simulink model "engine_with_auto_transmission_4spd_crcr"  (R2026a)
settings: Solver=VariableStepAuto  StopTime=15
libraries: nesl_utility x16, fl_lib x12, sdl_lib x9
settings Model: Creator=doyeop  LastModifiedBy=doyeop

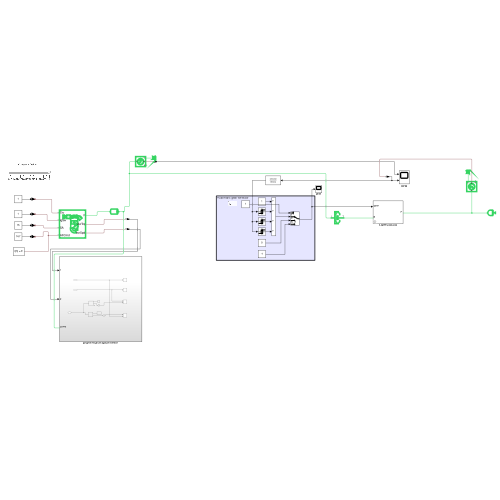
[thumbnail: Simulink's stored preview of the top-level diagram]
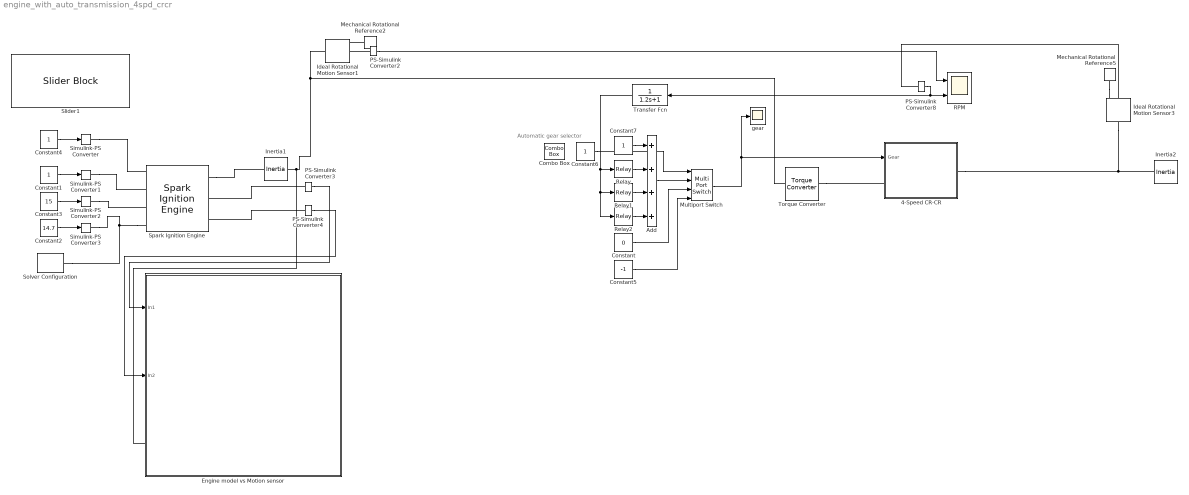
== system engine_with_auto_transmission_4spd_crcr ==
  note: Automatic gear selector
  4-Speed CR-CR : Subsystem  mask(4-Speed CR-CR){InitGear=Neutral, ShowInLibBrowser=0, ClutchSchedule={[0 1 1 0 0];[1 1 0 0 0];[1 0 1 0 0];[1 0 0 1 0];[0 0 0 1 1];[0 0 0 1 0]}}
      mask prompts: InitGear "Initial gear"
      mask help: physmod:sdl:library:transmissions:FourSpeedCRCR
      mask init:
      | set_param([gcb,'/Clutch A'],'initial_state_locked',num2str(ClutchSchedule{InitGear}(1)));
      | set_param([gcb,'/Clutch B'],'initial_state_locked',num2str(ClutchSchedule{InitGear}(2)));
      | set_param([gcb,'/Clutch C'],'initial_state_locked',num2str(ClutchSchedule{InitGear}(3)));
      | set_param([gcb,'/Clutch D'],'initial_state_locked',num2str(ClutchSchedule{InitGear}(4)));
      | set_param([gcb,'/Clutch R'],'initial_state_locked',num2str(ClutchSchedule{InitGear}(5)));
      mask Help: web([docroot '/sdl/ref/4speedcrcr.html'])
      mask TypeOptions InitGear: 4 | 3 | 2 | 1 | physmod:sdl:library:transmissions:Reverse | physmod:sdl:library:transmissions:Neutral
  Add : Sum  Inputs=++++
  Combo Box : ComboBox  LabelPosition=Hide  SelectedLabel=D
  Constant : Constant  Value=0
  Constant1 : Constant
  Constant2 : Constant  Value=14.7  SampleTime=-1
  Constant3 : Constant  Value=15  SampleTime=-1
  Constant4 : Constant  SampleTime=-1
  Constant5 : Constant  Value=-1
  Constant6 : Constant
  Constant7 : Constant
  Engine model vs Motion sensor : Subsystem
  Ideal Rotational Motion Sensor1 : fl_lib/Mechanical/Mechanical Sensors/Ideal Rotational Motion Sensor  reference=foundation.enum.MeasurementReference.difference  acceleration_port=false  velocity_port=true  position_port=true  wrap_angle=false  offset=0 rad
  Ideal Rotational Motion Sensor3 : fl_lib/Mechanical/Mechanical Sensors/Ideal Rotational Motion Sensor  reference=foundation.enum.MeasurementReference.difference  acceleration_port=false  velocity_port=true  position_port=true  wrap_angle=false  offset=0 rad
  Inertia1 : fl_lib/Mechanical/Rotational Elements/Inertia  inertia=0.7 kg*m^2  num_ports=foundation.enum.numPorts2.two  w_specify=on  w_priority=High  w=1200 rpm  w_nominal_specify=off  w_nominal_value=1  w_nominal_unit=rad/s  t_specify=off  t_priority=None  t=0 N*m  t_nominal_specify=off  t_nominal_value=1  t_nominal_unit=N*m
  Inertia2 : fl_lib/Mechanical/Rotational Elements/Inertia  inertia=0.5 kg*m^2  num_ports=foundation.enum.numPorts2.one  w_specify=on  w_priority=None  w=0 rpm  w_nominal_specify=off  w_nominal_value=1  w_nominal_unit=rad/s  t_specify=off  t_priority=None  t=0 N*m  t_nominal_specify=off  t_nominal_value=1  t_nominal_unit=N*m
  Mechanical Rotational Reference2 : fl_lib/Mechanical/Rotational Elements/Mechanical Rotational Reference
  Mechanical Rotational Reference5 : fl_lib/Mechanical/Rotational Elements/Mechanical Rotational Reference
  Multiport Switch : MultiPortSwitch  DataPortOrder=Specify indices  DataPortIndices={1,0,-1}  SaturateOnIntegerOverflow=off  InputSameDT=off
  PS-Simulink Converter2 : nesl_utility/PS-Simulink Converter  PhysicalDomain=network_engine_domain  SubClassName=ps_output  LeftPortType=input  RightPortType=output  PseudoPeriodic=off  Frequencies=[]  VectorFormat=inherit  Unit=rpm  AffineConversion=off
  PS-Simulink Converter3 : nesl_utility/PS-Simulink Converter  PhysicalDomain=network_engine_domain  SubClassName=ps_output  LeftPortType=input  RightPortType=output  PseudoPeriodic=off  Frequencies=[]  VectorFormat=inherit  Unit=N*m  AffineConversion=off
  PS-Simulink Converter4 : nesl_utility/PS-Simulink Converter  PhysicalDomain=network_engine_domain  SubClassName=ps_output  LeftPortType=input  RightPortType=output  PseudoPeriodic=off  Frequencies=[]  VectorFormat=inherit  Unit=rpm  AffineConversion=off
  PS-Simulink Converter8 : nesl_utility/PS-Simulink Converter  PhysicalDomain=network_engine_domain  SubClassName=ps_output  LeftPortType=input  RightPortType=output  PseudoPeriodic=off  Frequencies=[]  VectorFormat=inherit  Unit=rpm  AffineConversion=off
  RPM : Scope  NumInputPorts=2
      settings: ActiveDisplayYMinimum=-326.02351905011483  ActiveDisplayYMaximum=2934.21167144869  DataLoggingVariableName=ScopeData3
  Relay : Relay  OnSwitchValue=500  OffSwitchValue=300
  Relay1 : Relay  OnSwitchValue=750  OffSwitchValue=500
  Relay2 : Relay  OnSwitchValue=1500  OffSwitchValue=750
  Simulink-PS Converter : nesl_utility/Simulink-PS Converter  PhysicalDomain=network_engine_domain  SubClassName=ps_input  LeftPortType=input  RightPortType=output  PseudoPeriodic=off  Frequencies=[]  NoiseDistribution=none  NoiseParameters=[]  Unit=1  AffineConversion=off  FilteringAndDerivatives=provide  SimscapeFilterOrder=1  InputFilterTimeConstant=0.001  UdotUserProvided=0
  Simulink-PS Converter1 : nesl_utility/Simulink-PS Converter  PhysicalDomain=network_engine_domain  SubClassName=ps_input  LeftPortType=input  RightPortType=output  PseudoPeriodic=off  Frequencies=[]  NoiseDistribution=none  NoiseParameters=[]  Unit=1  AffineConversion=off  FilteringAndDerivatives=provide  SimscapeFilterOrder=1  InputFilterTimeConstant=0.001  UdotUserProvided=0
  Simulink-PS Converter2 : nesl_utility/Simulink-PS Converter  PhysicalDomain=network_engine_domain  SubClassName=ps_input  LeftPortType=input  RightPortType=output  PseudoPeriodic=off  Frequencies=[]  NoiseDistribution=none  NoiseParameters=[]  Unit=deg  AffineConversion=off  FilteringAndDerivatives=provide  SimscapeFilterOrder=1  InputFilterTimeConstant=0.001  UdotUserProvided=0
  Simulink-PS Converter3 : nesl_utility/Simulink-PS Converter  PhysicalDomain=network_engine_domain  SubClassName=ps_input  LeftPortType=input  RightPortType=output  PseudoPeriodic=off  Frequencies=[]  NoiseDistribution=none  NoiseParameters=[]  Unit=1  AffineConversion=off  FilteringAndDerivatives=provide  SimscapeFilterOrder=1  InputFilterTimeConstant=0.001  UdotUserProvided=0
  Slider1 : SliderBlock  ScaleMax=1
  Solver Configuration : nesl_utility/Solver Configuration  PhysicalDomain=network_engine_domain  SubClassName=solver  LeftPortType=input  RightPortType=generic  Tones=[]  Harmonics=[]  SimulateNoise=off  Profile=off  UseLocalSampling=off  EnableSwitchedLinearOptims=on  FrequencyDomain=off  UseCCode=off  RelTol=0.001  AbsTol=0.001  MinStep=1e-09  ToWorkspace=off  RevertToSquareIcSolve=off  NumHomotopyIterations=100  PhasorMode=off  PhasorModeNumHarmonics=1  ConsistencySolver=NEWTON_XTOL_AFTER_FTOL  CanonicalOrdering=CANONICAL  OptimizeIntermediates=OPTIMIZED  IndexReductionMethod=DerivativeReplacement  DoDC=off  ResidualTolerance=1e-09  ConsistencyTolSource=GLOBAL  ConsistencyAbsTol=0.001  ConsistencyRelTol=0.001  ConsistencyTolFactor=0.001  UseLocalSolver=off  LocalSolverChoice=NE_BACKWARD_EULER_ADVANCER  ResolveIndetEquations=on  FunctionEvalNumThread=1  LocalSolverSampleTime=0.001  DoFixedCost=off  MaxNonlinIter=3  MaxModeIter=2  ComputeImpulses=off  ImpulseIterations=2  LinearAlgebra=auto  LinearAlgebraNumThread=0  EquationFormulation=NE_TIME_EF  DelaysMemoryBudget=1024  AutomaticFiltering=on  FilteringTimeConstant=0.001  PartitionStorageMethod=AS_NEEDED  PartitionMemoryBudget=1024  PartitionMethod=ROBUST  MultibodyUseLocalSolver=off  MultibodyLocalSolverChoice=ODE1  MultibodyLocalSolverSampleTime=0.001
  Spark Ignition Engine : sdl_lib/Engines & Motors/Spark Ignition Engine  numCyls=sdl.enum.engineNumCylinders.Four  twoCylSADiff=270 deg  L4FiringOrder=sdl.enum.engineFiringOrderFourCylinders.L4_1342  bore=67 mm  stroke=42.5 mm  conrod=90 mm  CR=12.2  P_amb=101.325 kPa  T_amb=298.15 K  rho_air=1.225 mg/cm^3  R_air=288.1965 J/(K*kg)  UseAirIntake=true  c_thr=0.1 s  thr_rest=3 deg  D_plate=8 cm  S_leak=0.3 cm^2  V_im=500 cm^3  Cd_in=0.9  IVO_0=-10 deg  IVC_0=100 deg  EVO_0=30 deg  EVC_0=5 deg  UseInVVT=false  UseExVVT=false  q_LHV=44.3 MJ/kg  InputAFR=true  AFR_const=14.6  InputInjPw=false  Sinj=6.5 mg/ms  SparkInputType=sdl.enum.engineSparkInputType.Angle  SA_const=20 deg  comb_bd=50 deg  dt_Pcyl_slow_decay=60 s  dt_Tcyl_slow_decay=600 s  dt_exh_decay=5 ms  InputBackPressure=false  dP_exh=50 kPa  dw_exh=6000 rpm  UseExhaustThermal=true  S_exh=1 m^2  M_exh=5 kg  C_exh=100 J/(K*kg)  k_gas=10 s  h_convection=100 W/(K*m^2)  k_radiation=0.3  SB=5.7e-8 W/(K^4*m^2)  Pim_0=101.325 kPa  ca0=0 deg  w0=0 rpm  EngSpdSimLimit=16000 rpm  OutputTorqueAvr=true  OutputSpeedAvr=true  OutputCrkpos=false  OutputPim=false  OutputAirMassFlow=false  OutputFuelMassFlow=false  OutputAFR=false  OutputVcyl=false  OutputPcyl=false  OutputTcyl=false  OutputTexh=false
  Torque Converter : sdl_lib/Couplings & Drives/Torque Converter  coast_mode_modeling=sdl.enum.torqueConverterContinuousTwomode.twomode  SR_drive_tlu=[0, .5, .6, .7, .8, .87, .92, .94, .96, .97, 1]  TR_drive_tlu=[2.232, 1.5462, 1.4058, 1.2746, 1.1528, 1.0732, 1.0192, 1, 1, 1, 1]  CF_drive_tlu=1e-4 * [.72558, .66322, .63463, .59042, .51331, .4144, .29287, .22444, .12186, .04386, 0] N*m/rpm^2  SR_coast_tlu=[0, .5, .6, .7, .8, .87, .92, .94, .96, .97, 1]  CF_coast_tlu=1e-4 * [.5079, .4643, .4442, .4133, .3593, .2901, .205, .1571, .0853, .0307, 0] N*m/rpm^2  iniMode=sdl.enum.torqueConverterInitialMode.coast  delta_w=1 rpm  n_vector=[0, .5, .6, .7, .8, .87, .92, .94, .96, .97]  trq_vector=[2.232, 1.5462, 1.4058, 1.2746, 1.1528, 1.0732, 1.0192, .9983, .9983, .9983]  cf_vector_parameterization=sdl.enum.torqueConverterCFParameterization.SpeedToSqrtTorque  cf_vector_reference_speed=sdl.enum.torqueConverterCFReferenceSpeed.ImpellerSpeedAlways  cf_vector=[12.2938, 12.8588, 13.1452, 13.6285, 14.6163, 16.2675, 19.3503, 22.1046, 29.9986, 50] rad/(N^(1/2)*m^(1/2)*s)  cf_vector_sq=1e-3 * [6.616, 6.048, 5.787, 5.384, 4.681, 3.779, 2.671, 2.047, 1.111, .4] N*m*s^2/rad^2  interp_method=simscape.enum.interpolation.linear  extrap_method=simscape.enum.extrapolation.linear  model_lag=sdl.enum.torqueConverterLagOnOff.LagOff  tau=.02 s  initial_trq_ratio=0
  Transfer Fcn : TransferFcn  Denominator=[1.2 1]
  gear : Scope
      settings: ActiveDisplayYMinimum=0.62500000000000011  ActiveDisplayYMaximum=4.375  DataLoggingVariableName=ScopeData2
  wires:
  Constant2/1 -> Simulink-PS Converter3/1
  Constant3/1 -> Simulink-PS Converter2/1
  Constant4/1 -> Simulink-PS Converter/1
  Constant1/1 -> Simulink-PS Converter1/1
  PS-Simulink Converter2/1 -> RPM/1
  PS-Simulink Converter3/1 -> Engine model vs Motion sensor/1(In1)
  PS-Simulink Converter4/1 -> Engine model vs Motion sensor/2(In2)
  PS-Simulink Converter8/1 -> RPM/2, Transfer Fcn/1
  Constant6/1 -> Multiport Switch/1
  Constant/1 -> Multiport Switch/3
  Constant5/1 -> Multiport Switch/4
  Constant7/1 -> Add/1
  Relay/1 -> Add/2
  Relay1/1 -> Add/3
  Relay2/1 -> Add/4
  Add/1 -> Multiport Switch/2
  Multiport Switch/1 -> 4-Speed CR-CR/1(Gear), gear/1
  Transfer Fcn/1 -> Relay/1, Relay1/1, Relay2/1
  connections:
  Spark Ignition Engine/LConn4 -- Simulink-PS Converter3/RConn1 -- Solver Configuration/RConn1
  Simulink-PS Converter2/RConn1 -- Spark Ignition Engine/LConn3
  Simulink-PS Converter1/RConn1 -- Spark Ignition Engine/LConn2
  PS-Simulink Converter3/LConn1 -- Spark Ignition Engine/RConn2
  Simulink-PS Converter/RConn1 -- Spark Ignition Engine/LConn1
  Spark Ignition Engine/RConn1 -- Inertia1/RConn1
  PS-Simulink Converter4/LConn1 -- Spark Ignition Engine/RConn3
  PS-Simulink Converter2/LConn1 -- Ideal Rotational Motion Sensor1/RConn2
  Mechanical Rotational Reference2/LConn1 -- Ideal Rotational Motion Sensor1/RConn1
  Ideal Rotational Motion Sensor3/RConn2 -- PS-Simulink Converter8/LConn1
  Mechanical Rotational Reference5/LConn1 -- Ideal Rotational Motion Sensor3/RConn1
  Engine model vs Motion sensor/LConn1 -- Ideal Rotational Motion Sensor1/LConn1 -- Torque Converter/LConn1 -- Inertia1/LConn1
  Ideal Rotational Motion Sensor3/LConn1 -- 4-Speed CR-CR/RConn1 -- Inertia2/LConn1
  Torque Converter/RConn1 -- 4-Speed CR-CR/LConn1

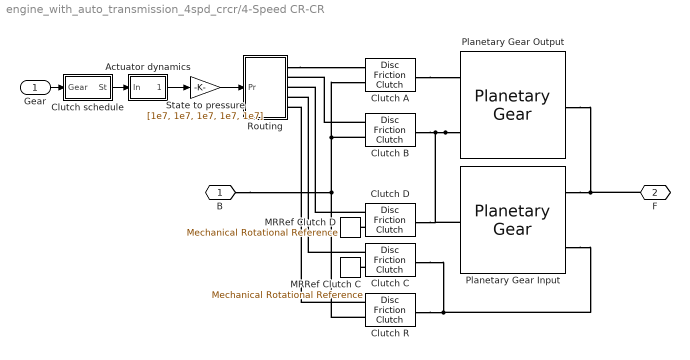
== system engine_with_auto_transmission_4spd_crcr/4-Speed CR-CR ==
  Gear : Inport
  Actuator dynamics : Subsystem  mask(First-order lag supporting vector signals){b=[1 1 1 1 1]*0.05, x_initial=ClutchSchedule{InitGear}}
      mask prompts: b "Filter time constant"; x_initial "Initial output"
      mask help: Models a lag of the form 1/(b*s+1) where s is the Laplace operator.
  Clutch schedule : Subsystem
  Clutch A : sdl_lib/Clutches/Disc Friction Clutch  geometry_model=1  r_eff=130 mm  d_o=0.15 m  d_i=0.1 m  nS=4  piston_area=0.001 m^2  unidirectional=0  friction_model=1  mu_w_vector=[ 0 0.1 0.2 0.3 0.4 0.5 1 2 5 10 100 1000 ] rad/s  temperature_TLU=[280.0, 300.0, 320.0] K  mu_static=.5  mu_static_vector=[0.4, 0.38, 0.36]  mu_coulomb=.5  mu_coulomb_vector=[ 0.29 0.28 0.26 0.22 0.21 0.2 0.2 0.19 0.19 0.19 0.19 0.19 ]  mu_coulomb_temp_vector=[0.3, 0.28, 0.25]  mu_coulomb_matrix=[0.34, 0.32, 0.3; 0.3, 0.28, 0.25; 0.25, 0.2, 0.15]  mu_interp_method=1  mu_extrap_method=1  d_f=1  w_tol=1e-3 rad/s  pressure_min=1e4 Pa  mu_visc=0 N*m/(rad/s)  initial_state_locked=0  thermal_mass=25 kJ/K  T_init=300 K
  Clutch B : sdl_lib/Clutches/Disc Friction Clutch  geometry_model=1  r_eff=130 mm  d_o=0.15 m  d_i=0.1 m  nS=4  piston_area=0.001 m^2  unidirectional=0  friction_model=1  mu_w_vector=[ 0 0.1 0.2 0.3 0.4 0.5 1 2 5 10 100 1000 ] rad/s  temperature_TLU=[280.0, 300.0, 320.0] K  mu_static=.5  mu_static_vector=[0.4, 0.38, 0.36]  mu_coulomb=.5  mu_coulomb_vector=[ 0.29 0.28 0.26 0.22 0.21 0.2 0.2 0.19 0.19 0.19 0.19 0.19 ]  mu_coulomb_temp_vector=[0.3, 0.28, 0.25]  mu_coulomb_matrix=[0.34, 0.32, 0.3; 0.3, 0.28, 0.25; 0.25, 0.2, 0.15]  mu_interp_method=1  mu_extrap_method=1  d_f=1  w_tol=1e-3 rad/s  pressure_min=1e4 Pa  mu_visc=0 N*m/(rad/s)  initial_state_locked=0  thermal_mass=25 kJ/K  T_init=300 K
  Clutch C : sdl_lib/Clutches/Disc Friction Clutch  geometry_model=1  r_eff=130 mm  d_o=0.15 m  d_i=0.1 m  nS=4  piston_area=0.001 m^2  unidirectional=0  friction_model=1  mu_w_vector=[ 0 0.1 0.2 0.3 0.4 0.5 1 2 5 10 100 1000 ] rad/s  temperature_TLU=[280.0, 300.0, 320.0] K  mu_static=.5  mu_static_vector=[0.4, 0.38, 0.36]  mu_coulomb=.5  mu_coulomb_vector=[ 0.29 0.28 0.26 0.22 0.21 0.2 0.2 0.19 0.19 0.19 0.19 0.19 ]  mu_coulomb_temp_vector=[0.3, 0.28, 0.25]  mu_coulomb_matrix=[0.34, 0.32, 0.3; 0.3, 0.28, 0.25; 0.25, 0.2, 0.15]  mu_interp_method=1  mu_extrap_method=1  d_f=1  w_tol=1e-3 rad/s  pressure_min=1e4 Pa  mu_visc=0 N*m/(rad/s)  initial_state_locked=0  thermal_mass=25 kJ/K  T_init=300 K
  Clutch D : sdl_lib/Clutches/Disc Friction Clutch  geometry_model=1  r_eff=130 m  d_o=0.15 m  d_i=0.1 m  nS=4  piston_area=0.001 m^2  unidirectional=0  friction_model=1  mu_w_vector=[ 0 0.1 0.2 0.3 0.4 0.5 1 2 5 10 100 1000 ] rad/s  temperature_TLU=[280.0, 300.0, 320.0] K  mu_static=.5  mu_static_vector=[0.4, 0.38, 0.36]  mu_coulomb=.5  mu_coulomb_vector=[ 0.29 0.28 0.26 0.22 0.21 0.2 0.2 0.19 0.19 0.19 0.19 0.19 ]  mu_coulomb_temp_vector=[0.3, 0.28, 0.25]  mu_coulomb_matrix=[0.34, 0.32, 0.3; 0.3, 0.28, 0.25; 0.25, 0.2, 0.15]  mu_interp_method=1  mu_extrap_method=1  d_f=1  w_tol=1e-3 rad/s  pressure_min=1e4 Pa  mu_visc=0 N*m/(rad/s)  initial_state_locked=1  thermal_mass=25 kJ/K  T_init=300 K
  Clutch R : sdl_lib/Clutches/Disc Friction Clutch  geometry_model=1  r_eff=130 mm  d_o=0.15 m  d_i=0.1 m  nS=4  piston_area=0.001 m^2  unidirectional=0  friction_model=1  mu_w_vector=[ 0 0.1 0.2 0.3 0.4 0.5 1 2 5 10 100 1000 ] rad/s  temperature_TLU=[280.0, 300.0, 320.0] K  mu_static=.5  mu_static_vector=[0.4, 0.38, 0.36]  mu_coulomb=.5  mu_coulomb_vector=[ 0.29 0.28 0.26 0.22 0.21 0.2 0.2 0.19 0.19 0.19 0.19 0.19 ]  mu_coulomb_temp_vector=[0.3, 0.28, 0.25]  mu_coulomb_matrix=[0.34, 0.32, 0.3; 0.3, 0.28, 0.25; 0.25, 0.2, 0.15]  mu_interp_method=1  mu_extrap_method=1  d_f=1  w_tol=1e-3 rad/s  pressure_min=1e4 Pa  mu_visc=0 N*m/(rad/s)  initial_state_locked=0  thermal_mass=25 kJ/K  T_init=300 K
  MRRef Clutch C : fl_lib/Mechanical/Rotational Elements/Mechanical Rotational Reference
  MRRef Clutch D : fl_lib/Mechanical/Rotational Elements/Mechanical Rotational Reference
  Planetary Gear Input : sdl_lib/Gears/Planetary Gear  rs_ratio=1.4  friction_model=1  efficiency=[ 0.96 0.98 ]  temperature_TLU=[ 280 300 320 ] K  efficiency_sp_TLU=[ 0.95 0.9 0.85 ]  efficiency_rp_TLU=[ 0.95 0.9 0.85 ]  pwr_thr=[ 0.001 0.001 ] W  mu_visc=[ 0 0 ] N*m/(rad/s)  model_inertia=true  sun_inertia=1e-10 kg*m^2  ring_inertia=1e-10 kg*m^2  carrier_inertia=1e-10 kg*m^2  carrier_radius=0.01 m  planet_inertia=0.001 kg*m^2  planet_mass=1e-10 kg  thermal_mass=50 J/K  T_init=300 K
  Planetary Gear Output : sdl_lib/Gears/Planetary Gear  rs_ratio=3.4  friction_model=1  efficiency=[ 0.96 0.98 ]  temperature_TLU=[ 280 300 320 ] K  efficiency_sp_TLU=[ 0.95 0.9 0.85 ]  efficiency_rp_TLU=[ 0.95 0.9 0.85 ]  pwr_thr=[ 0.001 0.001 ] W  mu_visc=[0 0] N*m/(rad/s)  model_inertia=true  sun_inertia=1e-10 kg*m^2  ring_inertia=1e-10 kg*m^2  carrier_inertia=1e-10 kg*m^2  carrier_radius=0.01 m  planet_inertia=0.001 kg*m^2  planet_mass=1e-10 kg  thermal_mass=50 J/K  T_init=300 K
  Routing : Subsystem
  State to pressure : Gain  Gain=[1e7, 1e7, 1e7, 1e7, 1e7]
  B : PMIOPort  Side=Left
  F : PMIOPort  Port=2  Side=Right
  wires:
  Actuator dynamics/1(Out) -> State to pressure/1
  Clutch schedule/1(St) -> Actuator dynamics/1(In)
  State to pressure/1 -> Routing/1(Pr)
  Gear/1 -> Clutch schedule/1(Gear)
  connections:
  Clutch R/RConn1 -- Planetary Gear Input/RConn2 -- Clutch C/RConn1
  Planetary Gear Output/RConn1 -- Planetary Gear Input/LConn1 -- Clutch D/RConn1 -- Clutch B/RConn1
  Planetary Gear Input/RConn1 -- Planetary Gear Output/LConn1 -- F/RConn1
  Clutch A/RConn1 -- Planetary Gear Output/RConn2
  Clutch R/LConn2 -- Clutch A/LConn2 -- Clutch B/LConn2 -- B/RConn1
  Routing/RConn1 -- Clutch A/LConn1
  Clutch D/LConn2 -- MRRef Clutch D/LConn1
  Clutch B/LConn1 -- Routing/RConn2
  Clutch C/LConn1 -- Routing/RConn4
  Clutch D/LConn1 -- Routing/RConn3
  Clutch C/LConn2 -- MRRef Clutch C/LConn1
  Clutch R/LConn1 -- Routing/RConn5

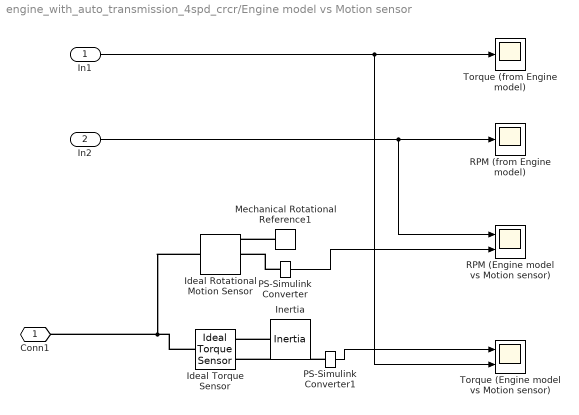
== system engine_with_auto_transmission_4spd_crcr/Engine model vs Motion sensor ==
  In1 : Inport
  In2 : Inport  Port=2
  Ideal Rotational Motion Sensor : fl_lib/Mechanical/Mechanical Sensors/Ideal Rotational Motion Sensor  reference=foundation.enum.MeasurementReference.difference  acceleration_port=false  velocity_port=true  position_port=true  wrap_angle=false  offset=0 rad
  Ideal Torque Sensor : fl_lib/Mechanical/Mechanical Sensors/Ideal Torque Sensor
  Inertia : fl_lib/Mechanical/Rotational Elements/Inertia  inertia=0.1 kg*m^2  num_ports=foundation.enum.numPorts2.one  w_specify=on  w_priority=None  w=0 rpm  w_nominal_specify=off  w_nominal_value=1  w_nominal_unit=rad/s  t_specify=off  t_priority=None  t=0 N*m  t_nominal_specify=off  t_nominal_value=1  t_nominal_unit=N*m
  Mechanical Rotational Reference1 : fl_lib/Mechanical/Rotational Elements/Mechanical Rotational Reference
  PS-Simulink Converter : nesl_utility/PS-Simulink Converter  PhysicalDomain=network_engine_domain  SubClassName=ps_output  LeftPortType=input  RightPortType=output  PseudoPeriodic=off  Frequencies=[]  VectorFormat=inherit  Unit=rpm  AffineConversion=off
  PS-Simulink Converter1 : nesl_utility/PS-Simulink Converter  PhysicalDomain=network_engine_domain  SubClassName=ps_output  LeftPortType=input  RightPortType=output  PseudoPeriodic=off  Frequencies=[]  VectorFormat=inherit  Unit=N*m  AffineConversion=off
  RPM (Engine model vs Motion sensor) : Scope  NumInputPorts=2
      settings: ActiveDisplayYMinimum=-419.44946675369869  ActiveDisplayYMaximum=3775.0452007832891
  RPM (from Engine model) : Scope
      settings: ActiveDisplayYMinimum=-545.70228379071159  ActiveDisplayYMaximum=4911.3205541164052  DataLoggingVariableName=ScopeData6
  Torque (Engine model vs Motion sensor) : Scope  NumInputPorts=2
      settings: ActiveDisplayYMinimum=-41.551396950603035  ActiveDisplayYMaximum=102.79160135138113
  Torque (from Engine model) : Scope
      settings: ActiveDisplayYMinimum=-2.7967171219384035  ActiveDisplayYMaximum=25.170454097445635  DataLoggingVariableName=ScopeData5
  Conn1 : PMIOPort  Side=Left
  wires:
  PS-Simulink Converter/1 -> RPM (Engine model vs Motion sensor)/2
  In2/1 -> RPM (from Engine model)/1, RPM (Engine model vs Motion sensor)/1
  In1/1 -> Torque (Engine model vs Motion sensor)/2, Torque (from Engine model)/1
  PS-Simulink Converter1/1 -> Torque (Engine model vs Motion sensor)/1
  connections:
  PS-Simulink Converter1/LConn1 -- Ideal Torque Sensor/RConn2
  Mechanical Rotational Reference1/LConn1 -- Ideal Rotational Motion Sensor/RConn1
  PS-Simulink Converter/LConn1 -- Ideal Rotational Motion Sensor/RConn2
  Ideal Torque Sensor/LConn1 -- Ideal Rotational Motion Sensor/LConn1 -- Conn1/RConn1
  Inertia/LConn1 -- Ideal Torque Sensor/RConn1

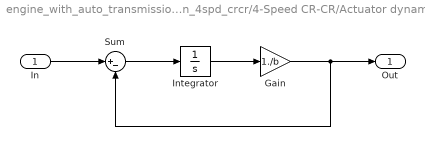
== system engine_with_auto_transmission_4spd_crcr/4-Speed CR-CR/Actuator dynamics ==
  In : Inport
  Gain : Gain  Gain=1./b
  Integrator : Integrator  InitialCondition=x_initial.*b
  Sum : Sum  Inputs=|+-  InputSameDT=on  SaturateOnIntegerOverflow=on  OutDataTypeStr=Inherit: Same as first input
  Out : Outport  VectorParamsAs1DForOutWhenUnconnected=off
  wires:
  Sum/1 -> Integrator/1
  In/1 -> Sum/1
  Integrator/1 -> Gain/1
  Gain/1 -> Sum/2, Out/1

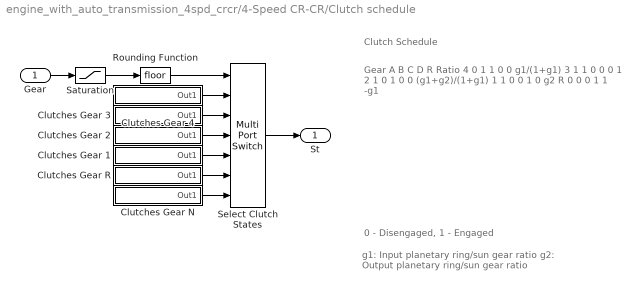
== system engine_with_auto_transmission_4spd_crcr/4-Speed CR-CR/Clutch schedule ==
  note: Gear
      | A
      | B
      | C
      | D
      | R
      | Ratio
      |
      | 4
      | 0
      | 1
      | 1
      | 0
      | 0
      | g1/(1+g1)
      |
      | 3
      | 1
      | 1
      | 0
      | 0
      | 0
      | 1
      |
      | 2
      | 1
      | 0
      | 1
      | 0
      | 0
      | (g1+g2)/(1+g1)
      |
      | 1
      | 1
      | 0
      | 0
      | 1
      | 0
      | g2
      |
      | R
      | 0
      | 0
      | 0
      | 1
      | 1
      | -g1
  note: g1: Input planetary ring/sun gear ratio
      | g2: Output planetary ring/sun gear ratio
  note: 0 - Disengaged, 1 - Engaged
  note: Clutch Schedule
  Gear : Inport
  Clutches Gear 1 : Subsystem  mask{Clutches=ClutchSchedule{4}}
      settings: OpenFcn=open_system(gcb,'force');
      mask Display: disp(Clutches)
  Clutches Gear 2 : Subsystem  mask{Clutches=ClutchSchedule{3}}
      settings: OpenFcn=open_system(gcb,'force');
      mask Display: disp(Clutches)
  Clutches Gear 3 : Subsystem  mask{Clutches=ClutchSchedule{2}}
      settings: OpenFcn=open_system(gcb,'force');
      mask Display: disp(Clutches)
  Clutches Gear 4 : Subsystem  mask{Clutches=ClutchSchedule{1}}
      settings: OpenFcn=open_system(gcb,'force');
      mask Display: disp(Clutches)
  Clutches Gear N : Subsystem  mask{Clutches=ClutchSchedule{6}}
      settings: OpenFcn=open_system(gcb,'force');
      mask Display: disp(Clutches)
  Clutches Gear R : Subsystem  mask{Clutches=ClutchSchedule{5}}
      settings: OpenFcn=open_system(gcb,'force');
      mask Display: disp(Clutches)
  Rounding Function : Rounding
  Saturation : Saturate  UpperLimit=4  LowerLimit=-1  ZeroCross=off
  Select Clutch States : MultiPortSwitch  DataPortOrder=Specify indices  DataPortIndices={4,3,2,1,-1,0}  DiagnosticForDefault=None  SaturateOnIntegerOverflow=off  InputSameDT=off
  St : Outport  VectorParamsAs1DForOutWhenUnconnected=off
  wires:
  Select Clutch States/1 -> St/1
  Clutches Gear 4/1(Out1) -> Select Clutch States/2
  Clutches Gear 2/1(Out1) -> Select Clutch States/4
  Clutches Gear 1/1(Out1) -> Select Clutch States/5
  Clutches Gear N/1(Out1) -> Select Clutch States/7
  Clutches Gear R/1(Out1) -> Select Clutch States/6
  Clutches Gear 3/1(Out1) -> Select Clutch States/3
  Rounding Function/1 -> Select Clutch States/1
  Gear/1 -> Saturation/1
  Saturation/1 -> Rounding Function/1

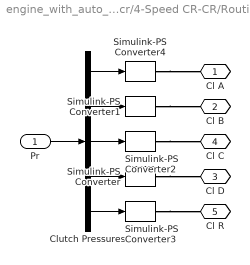
== system engine_with_auto_transmission_4spd_crcr/4-Speed CR-CR/Routing ==
  Pr : Inport
  Clutch Pressures : Demux  Outputs=5
  Simulink-PS Converter{,1..4} (5 alike) : nesl_utility/Simulink-PS Converter  PhysicalDomain=network_engine_domain  SubClassName=ps_input  LeftPortType=input  RightPortType=output  PseudoPeriodic=off  Frequencies=[]  NoiseDistribution=none  NoiseParameters=[]  Unit=1  AffineConversion=off  FilteringAndDerivatives=zero  SimscapeFilterOrder=1  InputFilterTimeConstant=.001  UdotUserProvided=0
  Cl A : PMIOPort  Side=Right
  Cl B : PMIOPort  Port=2  Side=Right
  Cl D : PMIOPort  Port=3  Side=Right
  Cl C : PMIOPort  Port=4  Side=Right
  Cl R : PMIOPort  Port=5  Side=Right
  wires:
  Clutch Pressures/1 -> Simulink-PS Converter4/1
  Clutch Pressures/3 -> Simulink-PS Converter2/1
  Clutch Pressures/5 -> Simulink-PS Converter3/1
  Clutch Pressures/2 -> Simulink-PS Converter1/1
  Clutch Pressures/4 -> Simulink-PS Converter/1
  Pr/1 -> Clutch Pressures/1
  connections:
  Simulink-PS Converter2/RConn1 -- Cl C/RConn1
  Simulink-PS Converter4/RConn1 -- Cl A/RConn1
  Simulink-PS Converter/RConn1 -- Cl D/RConn1
  Simulink-PS Converter1/RConn1 -- Cl B/RConn1
  Simulink-PS Converter3/RConn1 -- Cl R/RConn1

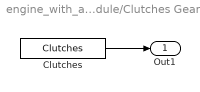
== system engine_with_auto_transmission_4spd_crcr/4-Speed CR-CR/Clutch schedule/Clutches Gear 1 ==
  Clutches : Constant  Value=Clutches  SampleTime=0
  Out1 : Outport  VectorParamsAs1DForOutWhenUnconnected=off
  wires:
  Clutches/1 -> Out1/1

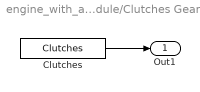
== system engine_with_auto_transmission_4spd_crcr/4-Speed CR-CR/Clutch schedule/Clutches Gear 2 ==
  Clutches : Constant  Value=Clutches  SampleTime=0
  Out1 : Outport  VectorParamsAs1DForOutWhenUnconnected=off
  wires:
  Clutches/1 -> Out1/1

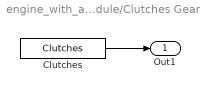
== system engine_with_auto_transmission_4spd_crcr/4-Speed CR-CR/Clutch schedule/Clutches Gear 3 ==
  Clutches : Constant  Value=Clutches  SampleTime=0
  Out1 : Outport  VectorParamsAs1DForOutWhenUnconnected=off
  wires:
  Clutches/1 -> Out1/1

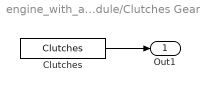
== system engine_with_auto_transmission_4spd_crcr/4-Speed CR-CR/Clutch schedule/Clutches Gear 4 ==
  Clutches : Constant  Value=Clutches  SampleTime=0
  Out1 : Outport  VectorParamsAs1DForOutWhenUnconnected=off
  wires:
  Clutches/1 -> Out1/1

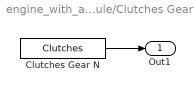
== system engine_with_auto_transmission_4spd_crcr/4-Speed CR-CR/Clutch schedule/Clutches Gear N ==
  Clutches Gear N : Constant  Value=Clutches  SampleTime=0
  Out1 : Outport  VectorParamsAs1DForOutWhenUnconnected=off
  wires:
  Clutches Gear N/1 -> Out1/1

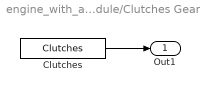
== system engine_with_auto_transmission_4spd_crcr/4-Speed CR-CR/Clutch schedule/Clutches Gear R ==
  Clutches : Constant  Value=Clutches  SampleTime=0
  Out1 : Outport  VectorParamsAs1DForOutWhenUnconnected=off
  wires:
  Clutches/1 -> Out1/1
